simulink model "HVDC_VSC_1CPUcore_dcpl"  (Simulink 8.4)
settings: Solver=ode3  SolverMode=SingleTasking  StartTime=0.0  StopTime=70.0  FixedStep=Ts_Power  RelTol=1e-3  AbsTol=1e-2
PreLoadFcn:
  | Ts_Power=50e-6; Ts_Control=1*Ts_Power; init_cosim_IA; startup_transients_hvdc_vsc;
PostLoadFcn:
  | Ts_Power=50e-6; Ts_Control=1*Ts_Power; init_cosim_IA; startup_transients_hvdc_vsc;
InitFcn:
  | Ts_Power=50e-6; Ts_Control=1*Ts_Power; init_cosim_IA; startup_transients_hvdc_vsc;
undefined symbols (not defined in the file): CLARK, D1, Delta, dPref1_2, dPref1_2_rlimit, gcbh, h, intfDelay, level, lib_mesures, magnitude, ResistanceM, rte_drive_private_lib, rte_tsb3level_hiz_rect_cb, sps_rtmsupport, t_deblock_Pref1, t_deblock_Udref2, t_dPref1_2, t_SwitchITMIdc, t_SwitchITMVdc, Ts_intf, TSB3_hiZR
libraries: powerlib x183, spsVIMeasurementModel x102, powerlib_extras x71, powerlib_meascontrol x50, rteventslib x26, op_dpl_lib x20, rtlab x14, sps_avr x6, artemis x1
(part 2 of 13)

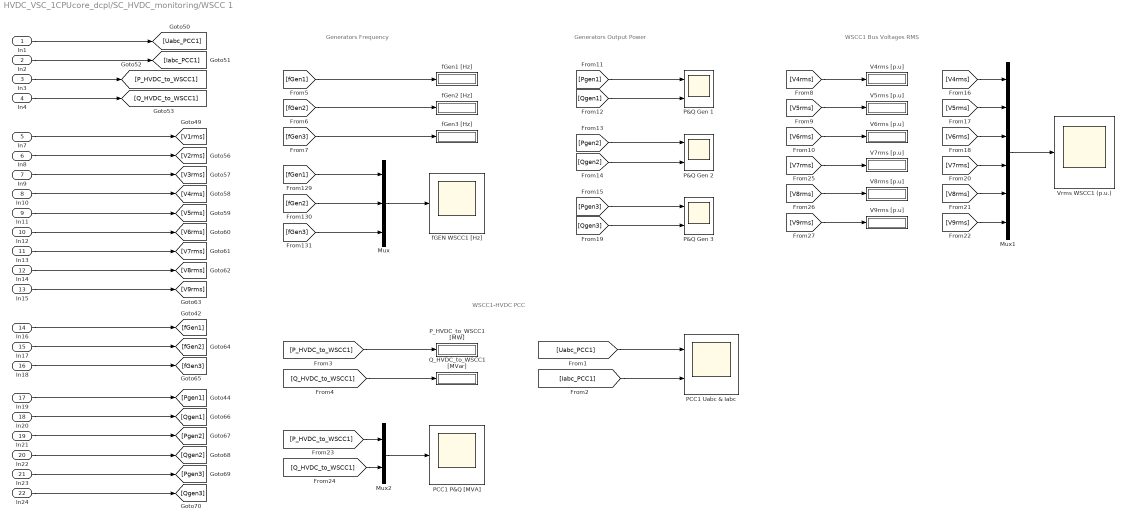
== system HVDC_VSC_1CPUcore_dcpl/SC_HVDC_monitoring/WSCC 1 ==
  note: Generators Frequency
  note: Generators Output Power
  note: WSCC1 Bus Voltages RMS
  note: WSCC1-HVDC PCC
  In1 : Inport
  In2 : Inport  Port=2
  In3 : Inport  Port=3
  In4 : Inport  Port=4
  In7 : Inport  Port=5
  In8 : Inport  Port=6
  In9 : Inport  Port=7
  In10 : Inport  Port=8
  In11 : Inport  Port=9
  In12 : Inport  Port=10
  In13 : Inport  Port=11
  In14 : Inport  Port=12
  In15 : Inport  Port=13
  In16 : Inport  Port=14
  In17 : Inport  Port=15
  In18 : Inport  Port=16
  In19 : Inport  Port=17
  In20 : Inport  Port=18
  In21 : Inport  Port=19
  In22 : Inport  Port=20
  In23 : Inport  Port=21
  In24 : Inport  Port=22
  Mux : Mux  Inputs=3
  Mux1 : Mux  Inputs=6
  Mux2 : Mux  Inputs=2
  P&Q Gen 1 : Scope  NumInputPorts=2
      settings: YMin=6e+07~-1.5e+08  YMax=2.2e+08~2e+08  SaveName=ScopeData19  Decimation=10
  P&Q Gen 2 : Scope  NumInputPorts=2
      settings: YMin=1.626e+08~5.9e+06  YMax=1.642e+08~6.7e+06  SaveName=ScopeData20  Decimation=10
  P&Q Gen 3 : Scope  NumInputPorts=2
      settings: YMin=8.46e+07~-1.115e+07  YMax=8.58e+07~-1.065e+07  SaveName=ScopeData22  Decimation=10
  PCC1 P&Q [MVA] : Scope
      settings: ShowLegends=on  YMin=-2.5e+08  YMax=2.5e+08  SaveName=ScopeData23  Decimation=10
  PCC1 Uabc & Iabc : Scope  NumInputPorts=2
      settings: ShowLegends=on  YMin=-2.5e+08~-5  YMax=2.5e+08~5  SaveName=ScopeData10  Decimation=10
  P_HVDC_to_WSCC1 [MW] : Display
  Q_HVDC_to_WSCC1 [MVar] : Display
  V4rms [p.u] : Display
  V5rms [p.u] : Display
  V6rms [p.u] : Display
  V7rms [p.u] : Display
  V8rms [p.u] : Display
  V9rms [p.u] : Display
  Vrms WSCC1 (p.u.) : Scope
      settings: ShowLegends=on  YMin=0.6  YMax=1.8  SaveName=ScopeData24  Decimation=10
  fGEN WSCC1 [Hz] : Scope
      settings: YMin=59.86  YMax=60  SaveName=ScopeData25  Decimation=10
  fGen1 [Hz] : Display
  fGen2 [Hz] : Display
  fGen3 [Hz] : Display
  wires:
  [Qgen2] -> P&Q Gen 2/2
  [Pgen2] -> P&Q Gen 2/1
  [Qgen3] -> P&Q Gen 3/2
  [Pgen3] -> P&Q Gen 3/1
  [Qgen1] -> P&Q Gen 1/2
  [Pgen1] -> P&Q Gen 1/1
  Mux/1 -> fGEN WSCC1 [Hz]/1
  In3/1 -> [P_HVDC_to_WSCC1]
  In10/1 -> [V4rms]
  In15/1 -> [V9rms]
  In12/1 -> [V6rms]
  [P_HVDC_to_WSCC1] -> Mux2/1
  In7/1 -> [V1rms]
  In13/1 -> [V7rms]
  In14/1 -> [V8rms]
  [V6rms] -> Mux1/3
  In8/1 -> [V2rms]
  [fGen1] -> Mux/1
  [V8rms] -> Mux1/5
  Mux2/1 -> PCC1 P&Q [MVA]/1
  In4/1 -> [Q_HVDC_to_WSCC1]
  [V4rms] -> Mux1/1
  In1/1 -> [Uabc_PCC1]
  [V5rms] -> Mux1/2
  In2/1 -> [Iabc_PCC1]
  In11/1 -> [V5rms]
  [V9rms] -> Mux1/6
  [V7rms] -> Mux1/4
  Mux1/1 -> Vrms WSCC1 (p.u.)/1
  [fGen2] -> Mux/2
  [fGen3] -> Mux/3
  In9/1 -> [V3rms]
  [Q_HVDC_to_WSCC1] -> Mux2/2
  In24/1 -> [Qgen3]
  In16/1 -> [fGen1]
  In23/1 -> [Pgen3]
  In19/1 -> [Pgen1]
  In18/1 -> [fGen3]
  In17/1 -> [fGen2]
  In20/1 -> [Qgen1]
  In21/1 -> [Pgen2]
  In22/1 -> [Qgen2]
  [Uabc_PCC1] -> PCC1 Uabc & Iabc/1
  [Iabc_PCC1] -> PCC1 Uabc & Iabc/2
  [fGen1] -> fGen1 [Hz]/1
  [fGen2] -> fGen2 [Hz]/1
  [fGen3] -> fGen3 [Hz]/1
  [V4rms] -> V4rms [p.u]/1
  [V5rms] -> V5rms [p.u]/1
  [V6rms] -> V6rms [p.u]/1
  [V7rms] -> V7rms [p.u]/1
  [V8rms] -> V8rms [p.u]/1
  [V9rms] -> V9rms [p.u]/1
  [P_HVDC_to_WSCC1] -> P_HVDC_to_WSCC1 [MW]/1
  [Q_HVDC_to_WSCC1] -> Q_HVDC_to_WSCC1 [MVar]/1

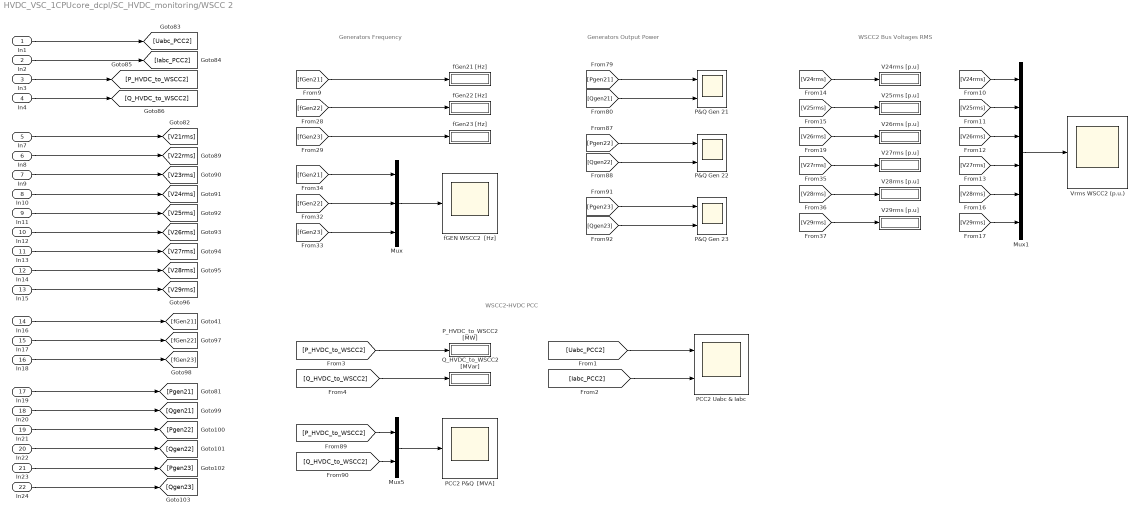
== system HVDC_VSC_1CPUcore_dcpl/SC_HVDC_monitoring/WSCC 2 ==
  note: Generators Frequency
  note: Generators Output Power
  note: WSCC2 Bus Voltages RMS
  note: WSCC2-HVDC PCC
  In1 : Inport
  In2 : Inport  Port=2
  In3 : Inport  Port=3
  In4 : Inport  Port=4
  In7 : Inport  Port=5
  In8 : Inport  Port=6
  In9 : Inport  Port=7
  In10 : Inport  Port=8
  In11 : Inport  Port=9
  In12 : Inport  Port=10
  In13 : Inport  Port=11
  In14 : Inport  Port=12
  In15 : Inport  Port=13
  In16 : Inport  Port=14
  In17 : Inport  Port=15
  In18 : Inport  Port=16
  In19 : Inport  Port=17
  In20 : Inport  Port=18
  In21 : Inport  Port=19
  In22 : Inport  Port=20
  In23 : Inport  Port=21
  In24 : Inport  Port=22
  Mux : Mux  Inputs=3
  Mux1 : Mux  Inputs=6
  Mux5 : Mux  Inputs=2
  P&Q Gen 21 : Scope  NumInputPorts=2
      settings: YMin=6e+07~-1.5e+08  YMax=2.2e+08~2e+08  SaveName=ScopeData8  Decimation=10
  P&Q Gen 22 : Scope  NumInputPorts=2
      settings: YMin=1.626e+08~5.9e+06  YMax=1.642e+08~6.7e+06  SaveName=ScopeData9  Decimation=10
  P&Q Gen 23 : Scope  NumInputPorts=2
      settings: YMin=8.46e+07~-1.115e+07  YMax=8.58e+07~-1.065e+07  SaveName=ScopeData11  Decimation=10
  PCC2 P&Q  [MVA] : Scope
      settings: ShowLegends=on  YMin=-1e+08  YMax=1.5e+08  SaveName=ScopeData13  Decimation=10
  PCC2 Uabc & Iabc : Scope  NumInputPorts=2
      settings: ShowLegends=on  YMin=-300000~-1000  YMax=300000~1500  SaveName=ScopeData14  Decimation=10
  P_HVDC_to_WSCC2 [MW] : Display
  Q_HVDC_to_WSCC2 [MVar] : Display
  V24rms [p.u] : Display
  V25rms [p.u] : Display
  V26rms [p.u] : Display
  V27rms [p.u] : Display
  V28rms [p.u] : Display
  V29rms [p.u] : Display
  Vrms WSCC2 (p.u.) : Scope
      settings: ShowLegends=on  YMin=0.6  YMax=1.8  SaveName=ScopeData27  Decimation=10
  fGEN WSCC2  [Hz] : Scope
      settings: YMin=59.86  YMax=60.02  SaveName=ScopeData28  Decimation=10
  fGen21 [Hz] : Display
  fGen22 [Hz] : Display
  fGen23 [Hz] : Display
  wires:
  In14/1 -> [V28rms]
  In20/1 -> [Qgen21]
  In3/1 -> [P_HVDC_to_WSCC2]
  In1/1 -> [Uabc_PCC2]
  In23/1 -> [Pgen23]
  [Qgen23] -> P&Q Gen 23/2
  [Qgen22] -> P&Q Gen 22/2
  [Pgen23] -> P&Q Gen 23/1
  [Pgen22] -> P&Q Gen 22/1
  [Qgen21] -> P&Q Gen 21/2
  [Q_HVDC_to_WSCC2] -> Mux5/2
  [P_HVDC_to_WSCC2] -> Mux5/1
  [Pgen21] -> P&Q Gen 21/1
  In18/1 -> [fGen23]
  In16/1 -> [fGen21]
  In21/1 -> [Pgen22]
  In9/1 -> [V23rms]
  In11/1 -> [V25rms]
  In17/1 -> [fGen22]
  In24/1 -> [Qgen23]
  In8/1 -> [V22rms]
  In13/1 -> [V27rms]
  In7/1 -> [V21rms]
  In4/1 -> [Q_HVDC_to_WSCC2]
  In19/1 -> [Pgen21]
  In22/1 -> [Qgen22]
  In10/1 -> [V24rms]
  In12/1 -> [V26rms]
  In15/1 -> [V29rms]
  In2/1 -> [Iabc_PCC2]
  [Uabc_PCC2] -> PCC2 Uabc & Iabc/1
  [Iabc_PCC2] -> PCC2 Uabc & Iabc/2
  Mux5/1 -> PCC2 P&Q  [MVA]/1
  Mux/1 -> fGEN WSCC2  [Hz]/1
  [V26rms] -> Mux1/3
  [fGen21] -> Mux/1
  [V28rms] -> Mux1/5
  [V24rms] -> Mux1/1
  [V25rms] -> Mux1/2
  [V29rms] -> Mux1/6
  [V27rms] -> Mux1/4
  Mux1/1 -> Vrms WSCC2 (p.u.)/1
  [fGen22] -> Mux/2
  [fGen23] -> Mux/3
  [fGen21] -> fGen21 [Hz]/1
  [fGen22] -> fGen22 [Hz]/1
  [fGen23] -> fGen23 [Hz]/1
  [V24rms] -> V24rms [p.u]/1
  [V25rms] -> V25rms [p.u]/1
  [V26rms] -> V26rms [p.u]/1
  [V27rms] -> V27rms [p.u]/1
  [V28rms] -> V28rms [p.u]/1
  [V29rms] -> V29rms [p.u]/1
  [P_HVDC_to_WSCC2] -> P_HVDC_to_WSCC2 [MW]/1
  [Q_HVDC_to_WSCC2] -> Q_HVDC_to_WSCC2 [MVar]/1

== system HVDC_VSC_1CPUcore_dcpl/SM_WSCC1_HVDCStation1/37.5-km  cable1 ==
  Artemis DPL1 : Subsystem
  Artemis DPL2 : Subsystem
  BI : Subsystem  Tag=ARTEMIS model
      settings: AttributesFormatString=%<Tag>
  PM1 : PMIOPort  Port=1  Side=Left
  PM2 : PMIOPort  Port=2  Side=Right
  wires:
  Artemis DPL1/1(ho) -> Artemis DPL2/1(hi)
  Artemis DPL2/1(ho) -> Artemis DPL1/1(hi)
  connections:
  PM1/RConn1 -- Artemis DPL1/LConn1
  Artemis DPL2/LConn1 -- PM2/RConn1

== system HVDC_VSC_1CPUcore_dcpl/SM_WSCC1_HVDCStation1/37.5-km cable1 ==
  Artemis DPL1 : Subsystem
  Artemis DPL2 : Subsystem
  BI : Subsystem  Tag=ARTEMIS model
      settings: AttributesFormatString=%<Tag>
  PM1 : PMIOPort  Port=1  Side=Left
  PM2 : PMIOPort  Port=2  Side=Right
  wires:
  Artemis DPL2/1(ho) -> Artemis DPL1/1(hi)
  Artemis DPL1/1(ho) -> Artemis DPL2/1(hi)
  connections:
  Artemis DPL2/LConn1 -- PM2/RConn1
  PM1/RConn1 -- Artemis DPL1/LConn1

== system HVDC_VSC_1CPUcore_dcpl/SM_WSCC1_HVDCStation1/B1 ==
  Kv : Gain  Gain=Ki  SaturateOnIntegerOverflow=on  OutDataTypeStr=Inherit: Same as input  ParamDataTypeStr=Inherit: Same as input
  Kv1 : Gain  Gain=Kv  SaturateOnIntegerOverflow=on  OutDataTypeStr=Inherit: Same as input  ParamDataTypeStr=Inherit: Same as input
  Mode I : spsVIMeasurementModel/Complex
  Mode V : spsVIMeasurementModel/Complex
  Model : spsVIMeasurementModel/VI  SystemSampleTime=-1
  A : PMIOPort  Port=1  Side=Left
  B : PMIOPort  Port=2  Side=Left
  C : PMIOPort  Port=3  Side=Left
  a : PMIOPort  Port=4  Side=Right
  b : PMIOPort  Port=5  Side=Right
  c : PMIOPort  Port=6  Side=Right
  tag scope: Iabc_B1=global, Uabc_B1=global
  wires:
  Model/2 -> Kv/1
  Model/1 -> Kv1/1
  Kv/1 -> Mode I/1
  Kv1/1 -> Mode V/1
  Mode I/1 -> [Iabc_B1]
  Mode V/1 -> [Uabc_B1]
  connections:
  Model/RConn3 -- c/RConn1
  Model/RConn1 -- a/RConn1
  Model/RConn2 -- b/RConn1
  Model/LConn3 -- C/RConn1
  Model/LConn1 -- A/RConn1
  Model/LConn2 -- B/RConn1

== system HVDC_VSC_1CPUcore_dcpl/SM_WSCC1_HVDCStation1/Station 1 (Rectifier) ==
  note: DC Capacitor
  note: Converter Station 1
  note: DC Filter
      | 3rd Harmonic
  note: Smoothing reactor
  200 MVA 230:100 kV 0.15 p.u. : powerlib/Elements/Three-Phase Transformer (Two Windings)  Winding1Connection=Yg  UNITS=pu  NominalPower=[200e6 , 60]  Winding1="[230e3 * 0.915  0.0025 0.075]"  Winding2Connection=Delta (D1)  Winding2="[100e3  0.0025  0.075]"  SetSaturation=off  Rm=500  Lm=500  Saturation=[ 0,0 ; 0.012,1.25 ; 1.012,1.6 ]  Hysteresis=off  DataFile='hysteresis'  SetInitialFlux=off  InitialFluxes=[-1.03850588171453 0.527233233676132 0.511272648041703]  Measurements=None  MoreParameters=off  BreakLoop=off  DataType=off  TransfoNumber=0
  A--> pu_AC_sec : Gain  Gain=1/(200e6/100e3/sqrt(3)*sqrt(2))
  Bconv1 : Subsystem  DialogController=POWERSYS.PowerSysDialog  LoadFcn=sps_rtmsupport('LoadFcn',gcbh);  StartFcn=sps_rtmsupport('StartFcn',gcbh);  StopFcn=sps_rtmsupport('StopFcn',gcbh);  mask(Three-Phase VI Measurement){VoltageMeasurement=phase-to-ground, SetLabelV=on, LabelV=Uv_abc1, Vpu=on, VpuLL=off, CurrentMeasurement=yes, SetLabelI=on, LabelI=Iv_abc1, Ipu=on, Pbase=200e6, Vbase=100e3, OutputType=Complex, PhasorSimulation=off, PSBequivalent=0}
      mask prompts: VoltageMeasurement "Voltage measurement"; SetLabelV "Use a label"; LabelV "Signal label  (use a From block to collect this signal)"; Vpu "Voltages in pu,  based on peak value of nominal phase-to-ground voltage"; VpuLL "Voltages in pu,  based on peak value of nominal phase-to-phase  voltage"; CurrentMeasurement "Current measurement"; SetLabelI "Use a label"; LabelI "Signal label  (use a From block to collect this signal)"; Ipu "Currents in pu"; Pbase "Base power ( VA 3 phase)"; Vbase "Nominal voltage used for pu measurement (Vrms phase-phase) :"; OutputType "Output signals in:"; PhasorSimulation "Phasor simulation (internal use)"; PSBequivalent "Equivalent circuit (internal use)"
      mask help:
      | Ideal three-phase voltage and current measurements.
      |
      | The block can output the voltages and currents in per unit values or in volts and amperes.
      mask init: same as HVDC_VSC_1CPUcore_dcpl/SM_WSCC1_HVDCStation1/B1
      settings: CopyFcn=sps_rtmsupport('CopyFcn',gcbh); powericon('ThreePhaseVIMeasurementCopy',gcb)  DeleteFcn=sps_rtmsupport('DeleteFcn',gcbh);  UndoDeleteFcn=sps_rtmsupport('UndoDeleteFcn',gcbh);  ModelCloseFcn=sps_rtmsupport('ModelCloseFcn',gcbh);  PreSaveFcn="sps_rtmsupport('PreSaveFcn',gcbh);  set_param(gcb,'LinkStatus','restore')"  PostSaveFcn=sps_rtmsupport('PostSaveFcn',gcbh);  NameChangeFcn=sps_rtmsupport('NameChangeFcn',gcbh);  PreCopyFcn=sps_rtmsupport('PreCopyFcn',gcbh);  OpenFcn=sps_rtmsupport('OpenFcn',gcbh, [1 2 4 5 6 7 9 -12 13]);  CloseFcn=sps_rtmsupport('CloseFcn',gcbh);  PreDeleteFcn=sps_rtmsupport('PreDeleteFcn',gcbh);
      mask Help: helpview(psbhelp)
      mask TypeOptions VoltageMeasurement: no | phase-to-ground | phase-to-phase
      mask Callback VoltageMeasurement: powericon('ThreePhaseVIMeasurementCback',gcb,'Vselector');
      mask Callback SetLabelV: powericon('ThreePhaseVIMeasurementCback',gcb,'');
      mask Callback Vpu: powericon('ThreePhaseVIMeasurementCback',gcb,'Vpu');
      mask Callback VpuLL: powericon('ThreePhaseVIMeasurementCback',gcb,'VpuLL');
      mask TypeOptions CurrentMeasurement: no | yes
      mask Callback CurrentMeasurement: powericon('ThreePhaseVIMeasurementCback',gcb,'');
      mask Callback SetLabelI: powericon('ThreePhaseVIMeasurementCback',gcb,'');
      mask Callback LabelI: powericon('ThreePhaseVIMeasurementCback',gcb,'');
      mask Callback Ipu: powericon('ThreePhaseVIMeasurementCback',gcb,'');
      mask TypeOptions OutputType: Complex | Real-Imag | Magnitude-Angle | Magnitude
  Bfilter1 : Subsystem  DialogController=POWERSYS.PowerSysDialog  LoadFcn=sps_rtmsupport('LoadFcn',gcbh);  StartFcn=sps_rtmsupport('StartFcn',gcbh);  StopFcn=sps_rtmsupport('StopFcn',gcbh);  mask(Three-Phase VI Measurement){VoltageMeasurement=phase-to-ground, SetLabelV=on, LabelV=Uf_abc1, Vpu=on, VpuLL=off, CurrentMeasurement=no, SetLabelI=off, LabelI=Iabc, Ipu=off, Pbase=100e6, Vbase=100e3, OutputType=Complex, PhasorSimulation=off, PSBequivalent=0}
      mask prompts: VoltageMeasurement "Voltage measurement"; SetLabelV "Use a label"; LabelV "Signal label  (use a From block to collect this signal)"; Vpu "Voltages in pu,  based on peak value of nominal phase-to-ground voltage"; VpuLL "Voltages in pu,  based on peak value of nominal phase-to-phase  voltage"; CurrentMeasurement "Current measurement"; SetLabelI "Use a label"; LabelI "Signal label  (use a From block to collect this signal)"; Ipu "Currents in pu"; Pbase "Base power ( VA 3 phase)"; Vbase "Nominal voltage used for pu measurement (Vrms phase-phase) :"; OutputType "Output signals in:"; PhasorSimulation "Phasor simulation (internal use)"; PSBequivalent "Equivalent circuit (internal use)"
      mask help:
      | Ideal three-phase voltage and current measurements.
      |
      | The block can output the voltages and currents in per unit values or in volts and amperes.
      mask init: same as HVDC_VSC_1CPUcore_dcpl/SM_WSCC1_HVDCStation1/B1
      settings: CopyFcn=sps_rtmsupport('CopyFcn',gcbh); powericon('ThreePhaseVIMeasurementCopy',gcb)  DeleteFcn=sps_rtmsupport('DeleteFcn',gcbh);  UndoDeleteFcn=sps_rtmsupport('UndoDeleteFcn',gcbh);  ModelCloseFcn=sps_rtmsupport('ModelCloseFcn',gcbh);  PreSaveFcn="sps_rtmsupport('PreSaveFcn',gcbh);  set_param(gcb,'LinkStatus','restore')"  PostSaveFcn=sps_rtmsupport('PostSaveFcn',gcbh);  NameChangeFcn=sps_rtmsupport('NameChangeFcn',gcbh);  PreCopyFcn=sps_rtmsupport('PreCopyFcn',gcbh);  OpenFcn=sps_rtmsupport('OpenFcn',gcbh, [1 2 4 5 6 7 9 -12 13]);  CloseFcn=sps_rtmsupport('CloseFcn',gcbh);  PreDeleteFcn=sps_rtmsupport('PreDeleteFcn',gcbh);
      mask Help: helpview(psbhelp)
      mask TypeOptions VoltageMeasurement: no | phase-to-ground | phase-to-phase
      mask Callback VoltageMeasurement: powericon('ThreePhaseVIMeasurementCback',gcb,'Vselector');
      mask Callback SetLabelV: powericon('ThreePhaseVIMeasurementCback',gcb,'');
      mask Callback Vpu: powericon('ThreePhaseVIMeasurementCback',gcb,'Vpu');
      mask Callback VpuLL: powericon('ThreePhaseVIMeasurementCback',gcb,'VpuLL');
      mask TypeOptions CurrentMeasurement: no | yes
      mask Callback CurrentMeasurement: powericon('ThreePhaseVIMeasurementCback',gcb,'');
      mask Callback SetLabelI: powericon('ThreePhaseVIMeasurementCback',gcb,'');
      mask Callback LabelI: powericon('ThreePhaseVIMeasurementCback',gcb,'');
      mask Callback Ipu: powericon('ThreePhaseVIMeasurementCback',gcb,'');
      mask TypeOptions OutputType: Complex | Real-Imag | Magnitude-Angle | Magnitude
  Cn1 : powerlib/Elements/Series RLC Branch  LConnTagsString=__new0  RConnTagsString=__new0  BranchType=C  Resistance=[]  Inductance=[]  SetiL0=off  InitialCurrent=0  Capacitance=70e-6  Setx0=off  InitialVoltage=0  Measurements=None
  Cn_DCF1 : powerlib/Elements/Series RLC Branch  LConnTagsString=__new0  RConnTagsString=__new0  BranchType=C  Resistance=[]  Inductance=[]  SetiL0=off  InitialCurrent=0  Capacitance=12e-6  Setx0=off  InitialVoltage=0  Measurements=None
  Cp1 : powerlib/Elements/Series RLC Branch  LConnTagsString=__new0  RConnTagsString=__new0  BranchType=C  Resistance=[]  Inductance=[]  SetiL0=off  InitialCurrent=0  Capacitance=70e-6  Setx0=off  InitialVoltage=0  Measurements=None
  Cp_DCF1 : powerlib/Elements/Series RLC Branch  LConnTagsString=__new0  RConnTagsString=__new0  BranchType=C  Resistance=[]  Inductance=[]  SetiL0=off  InitialCurrent=0  Capacitance=12e-6  Setx0=off  InitialVoltage=0  Measurements=None
  Current Measurement : powerlib/Measurements/Current Measurement  PhasorSimulation=off  OutputType=Complex  PSBequivalent=0
  Current Measurement1 : powerlib/Measurements/Current Measurement  PhasorSimulation=off  OutputType=Complex  PSBequivalent=0
  Filters 60Hz2 : Subsystem
      mask Display: disp('AC filters\n80 Mvar')
  L_DCF1 : powerlib/Elements/Series RLC Branch  LConnTagsString=__new0  RConnTagsString=__new0  BranchType=RL  Resistance=0.14737  Inductance=46.908e-3  SetiL0=off  InitialCurrent=0  Capacitance=[]  Setx0=off  InitialVoltage=0  Measurements=None
  Ln1 : powerlib/Elements/Series RLC Branch  LConnTagsString=__new0  RConnTagsString=__new0  BranchType=RL  Resistance=0.0251  Inductance=8.0e-3  SetiL0=off  InitialCurrent=0  Capacitance=[]  Setx0=off  InitialVoltage=0  Measurements=Branch current
  Lp1 : powerlib/Elements/Series RLC Branch  LConnTagsString=__new0  RConnTagsString=__new0  BranchType=RL  Resistance=0.0251  Inductance=8.0e-3  SetiL0=off  InitialCurrent=0  Capacitance=[]  Setx0=off  InitialVoltage=0  Measurements=Branch current
  Mux1 : Mux  Inputs=2
  Mux2 : Mux  Inputs=2
  Phase reactor 0.15 p.u. : powerlib/Elements/Three-Phase Series RLC Branch  LConnTagsString=A|B|C  RConnTagsString=A|B|C  BranchType=RL  Resistance=0.0015*(100^2 / 200)  Inductance=0.15* (100^2 / 200) / (2*pi*50)  Capacitance=1.0  Measurements=None
  TSB3_hiZR2 : Subsystem  AncestorBlock=rte_drive_private_lib/TSB3_hiZR  InitFcn=rte_tsb3level_hiz_rect_cb('InitFcn');  mask(3-Level TSB){legs=3, OutputType=Simulink double (mean model), Ron=0.0001, Vf=0, Ron_dio=0.0001, Vf_dio=0, NbMaxEvents=5, Rhi=2000, Snubber=0, Rsnu=22000, Common_mode_removal=off, dtct=1}
      mask prompts: legs "Number of bridge arms"; OutputType "Voltage output data type"; Ron "Active Switch Ron [ohms]"; Vf "Active Switch Forward voltage Vf [V]"; Ron_dio "Diode Ron [ohms]"; Vf_dio "Diode Forward voltage [V]"; NbMaxEvents "Maximum number of events"; Rhi "Hi impedance value (Ohms)"; Snubber "Emulate snubber effect"; Rsnu "Snubber Resistance Value"; Common_mode_removal "DC link current Common Mode Removal"; dtct "Dead Time current threshold (A)"
      mask help: The RTE-Drive 3-Level TSB block implements a 3-level bridge for which the gates are controlled by RTE signals.
      mask Help: eval('rte_help(''openhelp'',''RTE-Drive 3-Level Tsb'');');
      mask TypeOptions legs: 1 | 2 | 3
      mask TypeOptions OutputType: RT-Events RTE double (high precision model) | Simulink double (mean model) | SimPowerSystem PM (mean model)
      mask Display: plot([0 NaN 105 NaN 78.75 70.35 87.15 78.75 70.35 87.15 78.75 78.75 NaN 52.5 52.5 52.5 78.75 NaN 52.5 52.5 52.5 78.75 78.75 NaN 52.5 52.5 NaN 52.5 52.5 42 NaN 21 31.5 31.5 34.65 31.5 31.5],[0 NaN 111 NaN 59.94 46.62 46.62 59.94 59.94 59.94 59.94 73.26 NaN 99.9 74.37 74.37 74.37 NaN 11.1 33.3 33.3 33.3 46.62 NaN 74.37 63.27 NaN 33.3 44.4 55.5 NaN 49.95 49.95 53.28 49.95 46.62 49.95]);
  V--> pu_AC_sec : Gain  Gain=1/(100e3/sqrt(3)*sqrt(2))
  Voltage Measurement : powerlib/Measurements/Voltage Measurement  PhasorSimulation=off  OutputType=Complex  PSBequivalent=0
  Voltage Measurement1 : powerlib/Measurements/Voltage Measurement  PhasorSimulation=off  OutputType=Complex  PSBequivalent=0
  A : PMIOPort  Port=1  Side=Left
  B : PMIOPort  Port=2  Side=Left
  C : PMIOPort  Port=3  Side=Left
  Pos : PMIOPort  Tag=PMCPort  Port=4  Side=Right
  N : PMIOPort  Tag=PMCPort  Port=5  Side=Right
  Neg : PMIOPort  Tag=PMCPort  Port=6  Side=Right
  tag scope: IdcPN1=global, VdcPN1=global
  wires:
  Current Measurement/1 -> Mux2/1
  Current Measurement1/1 -> Mux2/2
  Mux2/1 -> A--> pu_AC_sec/1
  Voltage Measurement/1 -> Mux1/1
  Voltage Measurement1/1 -> Mux1/2
  Mux1/1 -> V--> pu_AC_sec/1
  V--> pu_AC_sec/1 -> [VdcPN1]
  A--> pu_AC_sec/1 -> [IdcPN1]
  [Pulses1] -> TSB3_hiZR2/1(g)
  connections:
  A/RConn1 -- 200 MVA 230:100 kV 0.15 p.u./LConn1
  B/RConn1 -- 200 MVA 230:100 kV 0.15 p.u./LConn2
  C/RConn1 -- 200 MVA 230:100 kV 0.15 p.u./LConn3
  Phase reactor 0.15 p.u./RConn1 -- Bconv1/LConn1
  Phase reactor 0.15 p.u./RConn2 -- Bconv1/LConn2
  Phase reactor 0.15 p.u./RConn3 -- Bconv1/LConn3
  TSB3_hiZR2/LConn3 -- Cn_DCF1/RConn1 -- Ln1/LConn1 -- Voltage Measurement1/LConn1 -- Cn1/RConn1
  TSB3_hiZR2/LConn1 -- Cp_DCF1/LConn1 -- Lp1/LConn1 -- Cp1/LConn1 -- Voltage Measurement/LConn1
  Current Measurement/RConn1 -- Pos/RConn1
  Current Measurement1/RConn1 -- Neg/RConn1
  200 MVA 230:100 kV 0.15 p.u./RConn1 -- Bfilter1/LConn1
  200 MVA 230:100 kV 0.15 p.u./RConn2 -- Bfilter1/LConn2
  200 MVA 230:100 kV 0.15 p.u./RConn3 -- Bfilter1/LConn3
  Bfilter1/RConn2 -- Filters 60Hz2/LConn2 -- Phase reactor 0.15 p.u./LConn2
  Bfilter1/RConn3 -- Filters 60Hz2/LConn3 -- Phase reactor 0.15 p.u./LConn3
  Phase reactor 0.15 p.u./LConn1 -- Filters 60Hz2/LConn1 -- Bfilter1/RConn1
  Cp_DCF1/RConn1 -- Cn_DCF1/LConn1 -- L_DCF1/RConn1
  TSB3_hiZR2/LConn2 -- N/RConn1 -- L_DCF1/LConn1 -- Cn1/LConn1 -- Cp1/RConn1 -- Voltage Measurement/LConn2 -- Voltage Measurement1/LConn2
  Lp1/RConn1 -- Current Measurement/LConn1
  Ln1/RConn1 -- Current Measurement1/LConn1
  Bconv1/RConn1 -- TSB3_hiZR2/RConn1
  Bconv1/RConn2 -- TSB3_hiZR2/RConn2
  Bconv1/RConn3 -- TSB3_hiZR2/RConn3

== system HVDC_VSC_1CPUcore_dcpl/SM_WSCC1_HVDCStation1/VSC Controller (Station 1) ==
  note: |-----------------------Ts_Control-----------------------|
  note: |------------Ts_Power------------|
  note: Sample time:
  note: |----------------Ts_Power--------------|
  note: Reference Steps
  note: VSC Controller
      | (Station 1)
  note: RTE Firing Pulse unit
  2*pi1 : Gain  Gain=2*pi  SaturateOnIntegerOverflow=on  OutDataTypeStr=Inherit: Same as input  ParamDataTypeStr=Inherit: Same as input
  3-level firing pulse unit for TSB : Subsystem  mask(3-phase RT-Event Discrete PWM Generator){Ts=Ts_Power}
      mask prompts: Ts "Sample time:"
  Anti-aliasing Filters : Subsystem  mask(Anti-aliasing (2nd order lowpass)){f0_aa=2000, Ts=Ts_Power}
      mask prompts: f0_aa "Cut-off frequency (Hz):"; Ts "Sample time:"
      mask init:
      | zeta = 1/sqrt(2);
  Block : Step  Time=t_deblock_Pref1  Before=1  After=0  SampleTime=Ts_Control
  Constant{1..2,4..6} (5 alike) : Constant  Value=0
  Constant3 : Constant  Value=0.0
  Discrete 3-phase PWM Generator : powerlib_extras/Discrete  Control Blocks/Discrete 3-phase PWM Generator  ModulatorType=3-level  ModulatorMode=Un-synchronized  nF=27  Fc=27*60  ModulatingSignals=off  m=0.86  Freq=50  Phase=-50  Ts=Ts_Power
  Discrete VSC Controller (Station 1) : Subsystem  mask(Discrete VSC-Based HVDC Controller){Mode=Active & Reactive Power, Xnom=[230e3, 100e3, 200e3, 200e6], XP=[20.0, 1.0, -1.0, 1.43], Xdvco=[3.0, 3.0, 1.05, 0.9], XUdc=[2.0, 40.0 ], XQ=[20.0, 0.5, -0.5], Xvco=[3.0, 3.0, 1.05, 0.94], Xcrc=[1.1,  0.8], Xaccc=[0.6, 6.0,  0.3], enable_dcvbc=off, Xdcvbc=[0.2, 0.03], Ts_Control=Ts_Control}
      mask prompts: Mode "Control Mode:"; Xnom "Nominal Voltages and Power: [ Vpcc(Vrms L-L) , Vconv (Vrms L-L),  Vdc (V L-L), Pnom (VA) ]"; XP "P Regulator [ Ki (1/s), Pmax (pu), Pmin (pu), Ramp (pu/s)]"; Xdvco "P Control: Udc Override [ Kp, Ki (1/s), Udc_max (pu), Udc_min (pu)]"; XUdc "DC Voltage Regulator [ Kp, Ki (1/s)]"; XQ "Q Regulator [ Ki (1/s), Qmax (pu), Qmin (pu)]"; Xvco "Q Control: Uac Override [ Kp, Ki (1/s), U_max (pu), U_min (pu)]"; Xcrc "Current Reference Limits [ lim_d (pu),  lim_q (pu)]"; Xaccc "Inner Current Regulator [ Kp, Ki (1/s), Kf (pu)]"; enable_dcvbc "DC Voltage Balance"; Xdcvbc "DC Voltage Balance Control} [ Kp, Ki (1/s)]"; Ts_Control "Sample Time (s)"
      mask help:
      | This block implements a controller for a VSC (Voltage-Sourced Converter) HVDC using a three-level or Neutral Point Clamped (NPC) converter bridge.
      | The 'Vref_abc' output contains the three modulating signals used by  the carrier-based  Sinusoidal Pulse Width Modulation (SPWM) pulse generator.
      | The output  'm' is a bus signal . Use the Bus Selector block to extract individual signals.
      |
      | See the "VSC-Based Transmission Link " tutorial for a description of the control system.
      mask init:
      | if (Mode == 1)
      | 	P_control = 1;
      | else
      | 	P_control = 0;
      | end
      | 	
      | % Nominal Voltages and Power:
      | VacNom1 = Xnom(1); VacNom2 = Xnom(2); VdcNom = Xnom(3); Pnom = Xnom(4);
      | % Normalisation Calculation
      | Uac_sec_to_pu   = 1/(VacNom2*sqrt(2)/sqrt(3));
      | k_nom2pu_Vdc = (VdcNom/2) * Uac_sec_to_pu;
      | k_pu2nom_Vdc = 1/k_nom2pu_Vdc;
      | k_nom2pu_Idc = ((VacNom2)*sqrt(3))/(sqrt(2)*VdcNom);
      | k_pu2nom_Idc = 1/k_nom2pu_Idc;
      | % Transformer connexion:
      | Tr_connection = 1;
      | % P regulator:
      | Ki_apc = XP(1); P_max = XP(2); P_min = XP(3); Ramp_apc = XP(4);
      | max_i_apc = 10; min_i_apc = -max_i_apc; V_level_apc = 0.9;  % (pu)
      | % DC Voltage Control Override:
      | Ki_apc_vco = Xdvco(2); Kp_apc_vco = Xdvco(1);
      | Udc_max = Xdvco(3)*k_nom2pu_Vdc; Udc_min = Xdvco(4)*k_nom2pu_Vdc;
      | max_apc_vco = 1.0; min_apc_vco = -max_apc_vco;
      | % Q regulator:
      | Ki_rpc = XQ(1);Q_max = XQ(2); Q_min = XQ(3);
      | max_i_rpc = 10; min_i_rpc = -max_i_rpc; V_level_rpc = 0.9;  % (pu)
      | % AC Voltage Control Override:
      | Ki_rpc_vco = Xvco(2); Kp_rpc_vco = Xvco(1);
      | U_max = Xvco(3); U_min = Xvco(4);
      | max_rpc_vco = 1.0; min_rpc_vco = -max_rpc_vco;
      | % Current Reference Calculation:
      | lim_d_crc = Xcrc(1); lim_q_crc = Xcrc(2); %(pu)
      | U_level_crc = 0.7; %(pu)
      | f0_crc = 120; % (Hz)
      | % Current Reference Limitation:
      | Iref_max = sqrt(lim_d_crc^2 + lim_q_crc^2);
      | % DC Voltage regulator:
      | Ki_dcvc = XUdc(2); Kp_dcvc = XUdc(1);
      | max_i_dcvc = lim_d_crc; min_i_dcvc = -max_i_dcvc;
      | max_out_dcvc = max_i_dcvc; min_out_dcvc = -max_out_dcvc; % (pu)
      | f0_Udc = 10.0; % (Hz)
      | % Inner Current Loop:
      | Ki_accc = Xaccc(2); Kp_accc = Xaccc(1); Kf_accc = Xaccc(3);
      | max_out_accc = 2.0; min_out_accc = -max_out_accc;
      | %PLL
      | f_min_pll = 55; % (Hz)
      | Kp_pll = 60.0;
      | Ki_pll = 1400;
      | % Inner Current Loop:
      | K_pwm = 1.0; 
      | % DC Voltage Balance Control:
      | Ki_dcvbc = Xdcvbc(2); Kp_dcvbc = Xdcvbc(1);
      | f0_dcvbc =  1.0;   % (Hz)
      | max_out_dcvbc = 0.2; min_out_dcvbc = -max_out_dcvbc;
      | % Signal Calculations:
      | f0_sc = 17; %(Hz)
      | zeta_sc = 1/sqrt(2);
      mask TypeOptions Mode: Active & Reactive Power | DC Voltage & Reactive  Power
      mask Callback Mode:
      | tempMaskVis=get_param(gcb,'MaskVisibilities');
      | if strcmp(get_param(gcb,'Mode'),'Active & Reactive Power')
      | 	tempMaskVis{2}='on'; tempMaskVis{3}='on'; tempMaskVis{4}='on'; tempMaskVis{5}='on';
      | 	tempMaskVis{6}='on'; tempMaskVis{5}='off'; tempMaskVis{8}='on'; tempMaskVis{9}='on';
      | 	tempMaskVis{10}='on';  tempMaskVis{12}='on';
      | 
      | else
      | 	tempMaskVis{2}='on'; tempMaskVis{3}='off'; tempMaskVis{4}='off'; tempMaskVis{5}='on';
      | 	tempMaskVis{6}='on'; tempMaskVis{7}='on'; tempMaskVis{8}='on'; tempMaskVis{9}='on';
      | 	tempMaskVis{10}='on';  tempMaskVis{12}='on';
      | end
      | if strcmp(get_param(gcb,'enable_dcvbc'),'on')
      | 	tempMaskVis{11}='on';
      | else
      | 	tempMaskVis{11}='off';
      | end
      | set_param(gcb,'MaskVisibilities',tempMaskVis);
      mask Callback enable_dcvbc:
      | tempMaskVis=get_param(gcb,'MaskVisibilities');
      | if strcmp(get_param(gcb,'enable_dcvbc'),'on')
      | 	tempMaskVis{11}='on';
      | else
      | 	tempMaskVis{11}='off';
      | end
      | set_param(gcb,'MaskVisibilities',tempMaskVis);
  Discrete-Time Integrator2 : DiscreteIntegrator  SampleTime=Ts_Power
  Rate Limiter : RateLimiter  RisingSlewLimit=dPref1_2_rlimit  FallingSlewLimit=-dPref1_2_rlimit  SampleTimeMode=inherited
  Sum3 : Sum  Inputs=+++  SaturateOnIntegerOverflow=on
  Switch : Switch  Threshold=0.5  SaturateOnIntegerOverflow=on
  Switch1 : Switch  Threshold=0.5  SaturateOnIntegerOverflow=on
  Switch2 : Switch  Threshold=0.5  SaturateOnIntegerOverflow=on
  Switching_Frequency : Constant  Value=27*60
  Terminator : Terminator
  Unit Delay : UnitDelay  SampleTime=Ts_Control
  Zero-Order Hold{1..3,5,7,13} (6 alike) : ZeroOrderHold  SampleTime=Ts_Control
  dPref2 : Step  Time=t_dPref1_2  After=dPref1_2  SampleTime=Ts_Control
  tag scope: Control1=global, Pulses1=global, Qref1=global, Udref1=global, Vref_abc1=global
  wires:
  Discrete VSC Controller (Station 1)/1(Vref_abc) -> [Vref_abc1], Unit Delay/1
  Discrete 3-phase PWM Generator/2 -> Terminator/1
  Zero-Order Hold13/1 -> Discrete VSC Controller (Station 1)/1(Uabc (pu))
  Zero-Order Hold1/1 -> Discrete VSC Controller (Station 1)/2(Iabc (pu))
  Zero-Order Hold3/1 -> Discrete VSC Controller (Station 1)/3(Uf_abc (pu))
  Zero-Order Hold2/1 -> Discrete VSC Controller (Station 1)/4(Iv_abc (pu))
  Zero-Order Hold5/1 -> Discrete VSC Controller (Station 1)/5(Udc_pn (pu))
  Zero-Order Hold7/1 -> Discrete VSC Controller (Station 1)/6(Idc_pn (pu))
  [Iabc_B1] -> Anti-aliasing Filters/2("Iabc ")
  [Uf_abc1] -> Anti-aliasing Filters/3("Uf_abc  ")
  [Iv_abc1] -> Anti-aliasing Filters/4("Iv_abc ")
  Anti-aliasing Filters/2(Iabc) -> Zero-Order Hold1/1
  Anti-aliasing Filters/3(Uf_abc) -> Zero-Order Hold3/1
  Anti-aliasing Filters/4(" Iv_abc") -> Zero-Order Hold2/1
  Anti-aliasing Filters/5("Udc_pn ") -> Zero-Order Hold5/1
  Anti-aliasing Filters/6(" Idc_pn") -> Zero-Order Hold7/1
  Constant2/1 -> Switch/1
  Constant1/1 -> Discrete VSC Controller (Station 1)/10(Udref), [Udref1]
  Constant6/1 -> [Qref1], Discrete VSC Controller (Station 1)/9(Qref)
  Constant3/1 -> Discrete VSC Controller (Station 1)/7(Pref)
  Discrete 3-phase PWM Generator/1 -> Switch/3
  Block/1 -> Discrete VSC Controller (Station 1)/11(block_status), Switch/2, Switch1/2
  [VdcPN1] -> Anti-aliasing Filters/5("Udc_pn  ")
  [IdcPN1] -> Anti-aliasing Filters/6("Idc_pn ")
  Discrete VSC Controller (Station 1)/2(m) -> [Control1]
  [Uabc_B1] -> Anti-aliasing Filters/1("Uabc ")
  Anti-aliasing Filters/1(Uabc) -> Zero-Order Hold13/1
  3-level firing pulse unit for TSB/1(duty) -> Switch1/3
  Constant5/1 -> Switch1/1
  Discrete-Time Integrator2/1 -> 3-level firing pulse unit for TSB/2(wt)
  2*pi1/1 -> Discrete-Time Integrator2/1
  Switching_Frequency/1 -> 2*pi1/1
  Switch2/1 -> [Pulses1]
  Switch/1 -> Switch2/1
  Switch1/1 -> Switch2/3
  Constant4/1 -> Switch2/2
  Unit Delay/1 -> Discrete 3-phase PWM Generator/1, 3-level firing pulse unit for TSB/1(3 phase output frequency)
  dPref2/1 -> Rate Limiter/1
  Sum3/1 -> Discrete VSC Controller (Station 1)/8(dPref)
  Rate Limiter/1 -> Sum3/2
